simulink library "RCAM"  (R2018b)
settings: Solver=ode45  StartTime=0.0  StopTime=10.0  RelTol=1e-3  EnableMultiTasking=on
values from neighbouring files (symbols this model uses):
  a0 = 15.212    [RCAM_SS_flat_earth_wind.m]
  a1 = -155.2    [RCAM_SS_flat_earth_wind.m]
  a2 = 609.2    [RCAM_SS_flat_earth_wind.m]
  a3 = -768.5    [RCAM_SS_flat_earth_wind.m]
  alpha_L0 = -11.5*pi/180    (= -0.200712863979)    [RCAM_SS_flat_earth_wind.m]
  alpha_switch = 14.5*(pi/180)    (= 0.253072741539)    [RCAM_SS_flat_earth_wind.m]
  cbar = 6.6    [RCAM_SS_flat_earth_wind.m]
  depsda = 0.25    [RCAM_SS_flat_earth_wind.m]
  Ib = m*[40.07 0 -2.0923 ... (first row only)    [RCAM_SS_flat_earth_wind.m]
  lt = 24.8    [RCAM_SS_flat_earth_wind.m]
  m = 120000    [RCAM_SS_flat_earth_wind.m]
  n = 5.5    [RCAM_SS_flat_earth_wind.m]
  S = 260    [RCAM_SS_flat_earth_wind.m]
  St = 64    [RCAM_SS_flat_earth_wind.m]
  Umax = 120000*9.81    (= 1177200)    [RCAM_SS_flat_earth_wind.m]
  Xac = 0.12*cbar    (= 0.792)    [RCAM_SS_flat_earth_wind.m]
  Xapt1 = 0    [RCAM_SS_flat_earth_wind.m]
  Xapt2 = 0    [RCAM_SS_flat_earth_wind.m]
  Yac = 0    [RCAM_SS_flat_earth_wind.m]
  Yapt1 = -7.94    [RCAM_SS_flat_earth_wind.m]
  Yapt2 = 7.94    [RCAM_SS_flat_earth_wind.m]
  Zac = 0    [RCAM_SS_flat_earth_wind.m]
  Zapt1 = -1.9    [RCAM_SS_flat_earth_wind.m]
  Zapt2 = -1.9    [RCAM_SS_flat_earth_wind.m]
undefined symbols (not defined in the file or in its folder): RCAM_SS_flat_earth_wind, X0, Xo
libraries: UWAerospaceBlockset_Utilities x4, $bdroot x3, aerolibutil x2, aerolibobsolete x1, aerolibadyn x1, UWAerospaceBlockset_FlightParameters x1
settings Model: Creator=Christopher  LastModifiedBy=Christopher
settings DataIOCC: LimitDataPoints=on  SaveFormat=Array
settings OptimizationCC: LifeSpan=inf
settings DebuggingCC: SolverPrmCheckMsg=warning  SFUnexpectedBacktrackingDiag=warning  SFNoUnconditionalDefaultTransitionDiag=warning  SFExecutionAtInitializationDiag=none
settings HardwareCC: ProdBitPerPointer=32  ProdBitPerSizeT=32  ProdBitPerPtrDiffT=32  ProdLargestAtomicFloat=None  ProdIntDivRoundTo=Undefined  ProdEndianess=Unspecified  ProdWordSize=32  ProdHWDeviceType=32-bit Generic
settings ModelReferenceCC: PropagateSignalLabelsOutOfModel=off
settings SFSimCC: SimUseLocalCustomCode=off
settings RTWCC: RTWUseLocalCustomCode=off
settings CodeAppCC: StateflowObjectComments=on
settings GRTTargetCC: TargetLangStandard=C89/C90 (ANSI)  GeneratePreprocessorConditionals=Disable all
settings ConfigComp: CovMetricSettings=dw  CovHtmlReporting=on  CovSaveCumulativeToWorkspaceVar=on  CovSaveSingleToWorkspaceVar=on  CovExternalEMLEnable=off  CovSFcnEnable=off

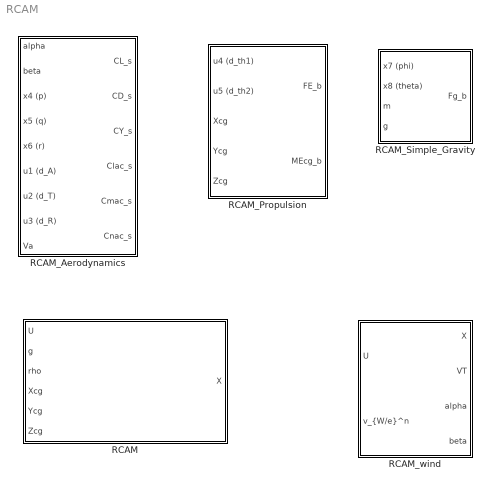
== system RCAM ==
  RCAM : Subsystem  mask{Xo=Xo, m=m, cbar=cbar, lt=lt, S=S, St=St, Xac=Xac, Yac=Yac, Zac=Zac, Umax=Umax, Xapt1=Xapt1, Yapt1=Yapt1, Zapt1=Zapt1, Xapt2=Xapt2, Yapt2=Yapt2, Zapt2=Zapt2, depsda=depsda, alpha_L0=alpha_L0, n=n, a3=a3, a2=a2, a1=a1, a0=a0, alpha_switch=alpha_switch, Ib=Ib}
      mask prompts: Xo "Xo: initial condition"; m "m: mass"; cbar "cbar: mean aerodynamic chord (m)"; lt "lt: distance bw AC of tail and body (m)"; S "S: wing planform area (m^2)"; St "St: tail planform area (m^2)"; Xac "Xac: x position of aerodynamic center in Fm (m)"; Yac "Yac: y position of aerodynamic center in Fm (m)"; Zac "Zac: z position of aerodynamic center in Fm (m)"; Umax "Umax: maximum thrust provided by one engine (N)"; Xapt1 "Xapt1: x position of engine 1 force in Fm (m)"; Yapt1 "Yapt1: y position of engine 1 force in Fm (m)"; Zapt1 "Zapt1: z position of engine 1 force in Fm (m)"; Xapt2 "Xapt2: x position of engine 2 force in Fm (m)"; Yapt2 "Yapt2: y position of engine 2 force in Fm (m)"; Zapt2 "Zapt2: z position of engine 2 force in Fm (m)"; depsda "depsda: change in downwash w.r.t. alpha (rad/rad)"; alpha_L0 "alpha_L0: zero lift angle of attack (rad)"; n "n: slope of linear region of lift slope"; alpha_switch "alpha_switch: alpha where lift slope goes from linear to non-linear"; Ib "Ib: inertia matrix"
      mask help:
      | Implements the RCAM model using Simulink blocks.
      |
      | State vector X and input vector U is defined as
      |
      |     X = [   u (m/s)
      |             v (m/s)
      |             w (m/s)
      |             p (rad/s)
      |             q (rad/s)
      |             r (rad/s)
      |             phi (bank angle: rad)
      |             theta (pitch angle: rad)
      |             psi (yaw angle: rad)
      |             P_N (position north (AKA X_e): m)
      |             P_E (position east (AKA Y_e): m)
      |             P_D (position down (AKA Z_e): m)
      |         ]
      |
      |     U = [   d_A (aileron deflection: rad)
      |             d_T (horizontal tail/elevator deflection: rad)
      |             d_R (rudder deflection: rad)
      |             d_th1 (throttle 1 deflection: in range [0,1])
      |             d_th2 (throttle 2 deflection: in range [0,1])
      |         ]
      |
      | The mass of this model is fixed but the CG location can move.
      |
      | INPUT:  U:      control vector
      |         g:      gravity magnitude (typically 9.81)
      |         rho:    density (kg/m^3)
      |         Xcg:    x position of CG (m)
      |         Ycg:    y position of CG (m)
      |         Zcg:    z position of CG (m)
      |
      | OUTPUT: X:      state vector
      |
      | Christopher Lum
      | lum@uw.edu
      mask Display: image('RCAM_icon.jpg')
  RCAM_Aerodynamics : Subsystem  mask{depsda=0.25, alpha_L0=-11.5*pi/180, n=5.5, a3=-768.5, a2=609.2, a1=-155.2, a0=15.2, alpha_switch=14.5*(pi/180), cbar=6.6, lt=24.8, S=260, St=64}
      mask prompts: depsda "depsda: change in downwash w.r.t. alpha (rad/rad)"; alpha_L0 "alpha_L0: zero lift angle of attack (rad)"; n "n: slope of linear region of lift slope"; alpha_switch "alpha_switch: alpha where lift slope goes from linear to non-linear (rad)"; cbar "cbar: mean aerodynamic chord"; lt "lt: distance between AC of tail and body"; S "S: wing planform area"; St "St: tail planform area"
      mask help:
      | Compute aerodynamic moment coefficients for the RCAM model.
      |
      | INPUT:  self explantory
      |
      | OUTPUT: force and moment coefficients such that the normalized values are expressed in the stability axis
  RCAM_Propulsion : Subsystem  mask{Umax=120000*9.81, Xapt1=0, Yapt1=-7.94, Zapt1=-1.9, Xapt2=0, Yapt2=7.94, Zapt2=-1.9}
      mask prompts: Umax "Umax (maximum engine thrust, same value applied to both engine 1 and 2)"; Xapt1 "Xapt1 (x position of engine 1 force in Fm)"; Yapt1 "Yapt1 (y position of engine 1 force in Fm)"; Zapt1 "Zapt1 (z position of engine 1 force in Fm)"; Xapt2 "Xapt2 (x position of engine 2 force in Fm)"; Yapt2 "Yapt2 (y position of engine 2 force in Fm)"; Zapt2 "Zapt2 (z position of engine 2 force in Fm)"
      mask help:
      | Calculates propulsion forces and moments for RCAM model.
      |
      | INPUT:  u4 (d_th1): throttle position 1
      |         u4 (d_th2): throttle position 2
      |         Xcg:        x location of CG
      |         Ycg:        y location of CG
      |         Zcg:        z location of CG
      |
      | OUTPUT: FE_b:       engine force vector expressed in body frame
      |         MEcg_b:     engine moment about CG expressed in body frame
  RCAM_Simple_Gravity : Subsystem
      mask help:
      | Computes the gravitational force in the body frame using the simple relationship of
      |
      | Fg_b = m*g*[-sin(x8);cos(x8)*sin(x7); cos(x8)*cos(x7)]
      |
      | INPUT:  x7 (phi):   bank Euler angle
      |         x8 (theta): pitch Euler angle
      |         m:          mass
      |         g:          gravitational acceleration
      |
      | OUTPUT: Fg_b:       gravitational force in body frame
  RCAM_wind : Subsystem  mask{Xo=X0}
      mask prompts: Xo "Xo: initial condition"
      mask help:
      | Implements the RCAM model with nominal constants with constant wind.
      |
      | State vector X and input vector U is defined as
      |
      |     X = [   u (m/s)
      |             v (m/s)
      |             w (m/s)
      |             p (rad/s)
      |             q (rad/s)
      |             r (rad/s)
      |             phi (bank angle: rad)
      |             theta (pitch angle: rad)
      |             psi (yaw angle: rad)
      |             P_N (position north (AKA X_e): m)
      |             P_E (position east (AKA Y_e): m)
      |             P_D (position down (AKA Z_e): m)
      |         ]
      |
      |     U = [   d_A (aileron deflection: rad)
      |             d_T (horizontal tail/elevator deflection: rad)
      |             d_R (rudder deflection: rad)
      |             d_th1 (throttle 1 deflection: in range [0,1])
      |             d_th2 (throttle 2 deflection: in range [0,1])
      |         ]
      |
      | The wind vector is defined as
      |
      |     v_{W/e}^n = [W_N; W_E; W_D]
      |
      | INPUT:  U:          control vector
      |         v_{W/e}^n:  3x1 wind vector
      |
      | OUTPUT: X:          state vector

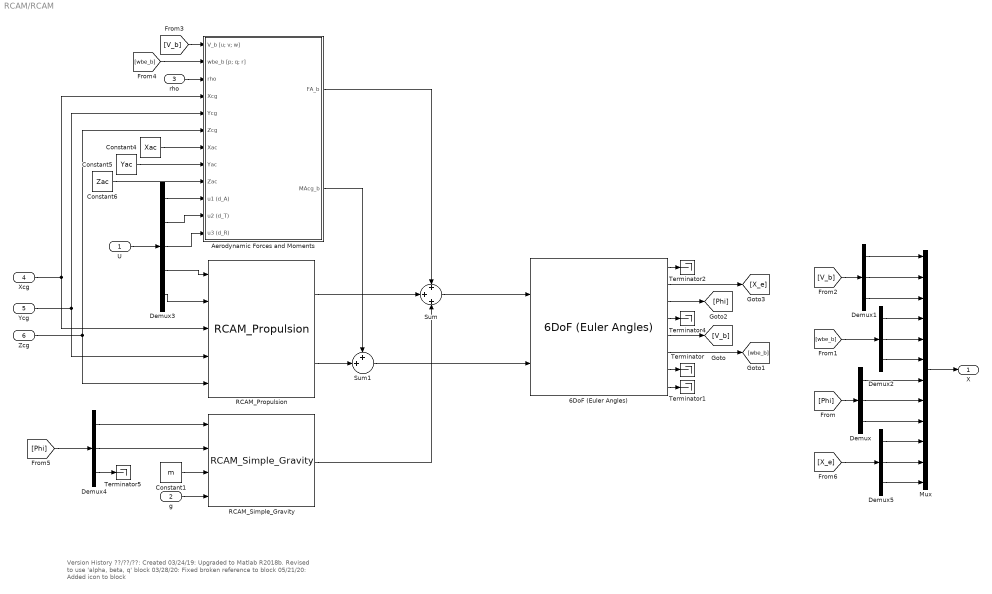
== system RCAM/RCAM ==
  note: Version History
      | ??/??/??: Created
      | 03/24/19: Upgraded to Matlab R2018b.  Revised to use 'alpha, beta, q' block
      | 03/28/20: Fixed broken reference to block
      | 05/21/20: Added icon to block
  U : Inport
  g : Inport  Port=2
  rho : Inport  Port=3
  Xcg : Inport  Port=4
  Ycg : Inport  Port=5
  Zcg : Inport  Port=6
  6DoF (Euler Angles) : aerolibobsolete/6DoF (Euler Angles)  units=Metric (MKS)  mtype=Fixed  rep=Euler Angles  xme_0=Xo(10:12)  Vm_0=Xo(1:3)  eul_0=Xo(7:9)  pm_0=Xo(4:6)  mass_0=m  mass_e=0.5  mass_f=2.0  inertia=Ib  inertia_e=eye(3)  inertia_f=2*eye(3)  k_quat=1.0
      settings: SourceProductName=Aerospace Blockset  SourceProductBaseCode=AE
  Aerodynamic Forces and Moments : Subsystem
  Constant1 : Constant  Value=m
  Constant4 : Constant  Value=Xac
  Constant5 : Constant  Value=Yac
  Constant6 : Constant  Value=Zac
  Demux{,1..2,4..5} (5 alike) : Demux  Outputs=3
  Demux3 : Demux  Outputs=5
  Mux : Mux  Inputs=12
  RCAM_Propulsion : $bdroot/RCAM_Propulsion  Umax=Umax  Xapt1=Xapt1  Yapt1=Yapt1  Zapt1=Zapt1  Xapt2=Xapt2  Yapt2=Yapt2  Zapt2=Zapt2
  RCAM_Simple_Gravity : $bdroot/RCAM_Simple_Gravity
  Sum : Sum  Inputs=+|+|+
  Sum1 : Sum  Inputs=++|
  Terminator{,1..2,4..5} (5 alike) : Terminator
  X : Outport
  wires:
  Aerodynamic Forces and Moments/1(FA_b) -> Sum/1
  RCAM_Propulsion/1 -> Sum/2
  RCAM_Simple_Gravity/1 -> Sum/3
  Aerodynamic Forces and Moments/2(MAcg_b) -> Sum1/1
  RCAM_Propulsion/2 -> Sum1/2
  Sum/1 -> 6DoF (Euler Angles)/1
  Sum1/1 -> 6DoF (Euler Angles)/2
  Demux/1 -> Mux/7
  Demux/2 -> Mux/8
  Demux/3 -> Mux/9
  Demux1/1 -> Mux/1
  Demux1/2 -> Mux/2
  Demux1/3 -> Mux/3
  Demux2/1 -> Mux/4
  Demux2/2 -> Mux/5
  Demux2/3 -> Mux/6
  6DoF (Euler Angles)/7 -> Terminator/1
  6DoF (Euler Angles)/8 -> Terminator1/1
  6DoF (Euler Angles)/1 -> Terminator2/1
  6DoF (Euler Angles)/2 -> [X_e]
  6DoF (Euler Angles)/4 -> Terminator4/1
  Mux/1 -> X/1
  6DoF (Euler Angles)/5 -> [V_b]
  6DoF (Euler Angles)/6 -> [wbe_b]
  6DoF (Euler Angles)/3 -> [Phi]
  [Phi] -> Demux/1
  [wbe_b] -> Demux2/1
  [V_b] -> Demux1/1
  rho/1 -> Aerodynamic Forces and Moments/3(rho)
  [V_b] -> Aerodynamic Forces and Moments/1(V_b [u; v; w])
  [wbe_b] -> Aerodynamic Forces and Moments/2(wbe_b [p; q; r])
  Constant4/1 -> Aerodynamic Forces and Moments/7(Xac)
  Constant5/1 -> Aerodynamic Forces and Moments/8(Yac)
  Constant6/1 -> Aerodynamic Forces and Moments/9(Zac)
  Demux3/1 -> Aerodynamic Forces and Moments/10(u1 (d_A))
  Demux3/2 -> Aerodynamic Forces and Moments/11(u2 (d_T))
  Demux3/3 -> Aerodynamic Forces and Moments/12(u3 (d_R))
  U/1 -> Demux3/1
  Demux3/4 -> RCAM_Propulsion/1
  Demux3/5 -> RCAM_Propulsion/2
  [Phi] -> Demux4/1
  Demux4/1 -> RCAM_Simple_Gravity/1
  Demux4/2 -> RCAM_Simple_Gravity/2
  Demux4/3 -> Terminator5/1
  Constant1/1 -> RCAM_Simple_Gravity/3
  g/1 -> RCAM_Simple_Gravity/4
  Xcg/1 -> RCAM_Propulsion/3, Aerodynamic Forces and Moments/4(Xcg)
  Ycg/1 -> RCAM_Propulsion/4, Aerodynamic Forces and Moments/5(Ycg)
  Zcg/1 -> RCAM_Propulsion/5, Aerodynamic Forces and Moments/6(Zcg)
  [X_e] -> Demux5/1
  Demux5/3 -> Mux/12
  Demux5/1 -> Mux/10
  Demux5/2 -> Mux/11

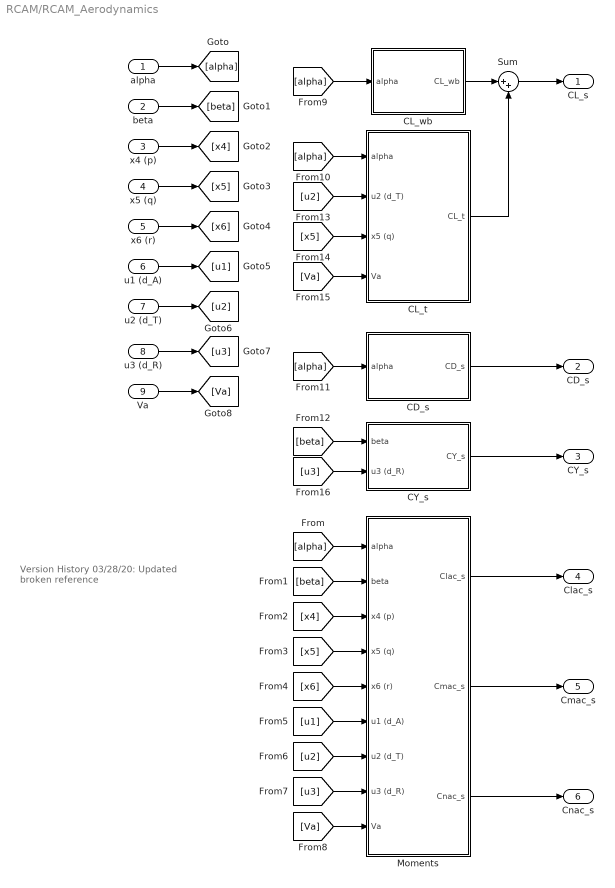
== system RCAM/RCAM_Aerodynamics ==
  note: Version History
      | 03/28/20: Updated broken reference
  alpha : Inport
  beta : Inport  Port=2
  x4 (p) : Inport  Port=3
  x5 (q) : Inport  Port=4
  x6 (r) : Inport  Port=5
  u1 (d_A) : Inport  Port=6
  u2 (d_T) : Inport  Port=7
  u3 (d_R) : Inport  Port=8
  Va : Inport  Port=9
  "CD_s " : Subsystem
  CL_t : Subsystem
  CL_wb : Subsystem
  "CY_s " : Subsystem
  Moments : Subsystem
  Sum : Sum  Inputs=|++
  CL_s : Outport
  CD_s : Outport  Port=2
  CY_s : Outport  Port=3
  Clac_s : Outport  Port=4
  Cmac_s : Outport  Port=5
  Cnac_s : Outport  Port=6
  wires:
  CL_wb/1(CL_wb) -> Sum/1
  CL_t/1(CL_t) -> Sum/2
  Sum/1 -> CL_s/1
  "CD_s "/1(CD_s) -> CD_s/1
  "CY_s "/1(CY_s) -> CY_s/1
  Moments/1(Clac_s) -> Clac_s/1
  Moments/2(Cmac_s) -> Cmac_s/1
  Moments/3(Cnac_s) -> Cnac_s/1
  alpha/1 -> [alpha]
  beta/1 -> [beta]
  x4 (p)/1 -> [x4]
  x5 (q)/1 -> [x5]
  x6 (r)/1 -> [x6]
  u1 (d_A)/1 -> [u1]
  u2 (d_T)/1 -> [u2]
  u3 (d_R)/1 -> [u3]
  Va/1 -> [Va]
  [alpha] -> Moments/1(alpha)
  [beta] -> Moments/2(beta)
  [x4] -> Moments/3(x4 (p))
  [x5] -> Moments/4(x5 (q))
  [x6] -> Moments/5(x6 (r))
  [u1] -> Moments/6(u1 (d_A))
  [u2] -> Moments/7(u2 (d_T))
  [u3] -> Moments/8(u3 (d_R))
  [Va] -> Moments/9(Va)
  [alpha] -> CL_wb/1(alpha)
  [alpha] -> CL_t/1(alpha)
  [alpha] -> "CD_s "/1(alpha)
  [beta] -> "CY_s "/1(beta)
  [u2] -> CL_t/2(u2 (d_T))
  [x5] -> CL_t/3(x5 (q))
  [Va] -> CL_t/4(Va)
  [u3] -> "CY_s "/2(u3 (d_R))

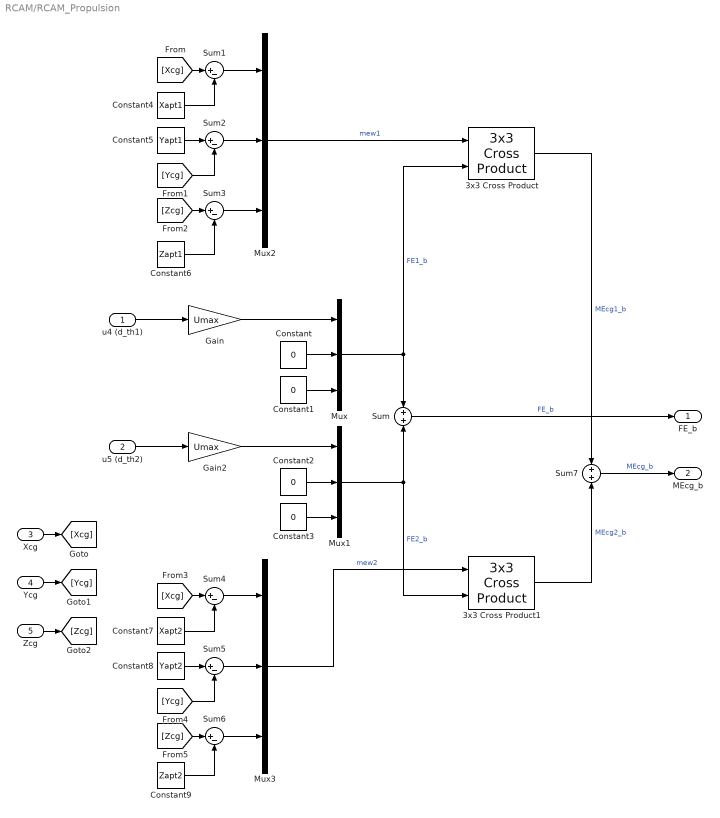
== system RCAM/RCAM_Propulsion ==
  u4 (d_th1) : Inport
  u5 (d_th2) : Inport  Port=2
  Xcg : Inport  Port=3
  Ycg : Inport  Port=4
  Zcg : Inport  Port=5
  3x3 Cross Product : aerolibutil/3x3 Cross Product
      settings: SourceProductName=Aerospace Blockset  SourceProductBaseCode=AE
  3x3 Cross Product1 : aerolibutil/3x3 Cross Product
      settings: SourceProductName=Aerospace Blockset  SourceProductBaseCode=AE
  Constant{,1..3} (4 alike) : Constant  Value=0
  Constant4 : Constant  Value=Xapt1
  Constant5 : Constant  Value=Yapt1
  Constant6 : Constant  Value=Zapt1
  Constant7 : Constant  Value=Xapt2
  Constant8 : Constant  Value=Yapt2
  Constant9 : Constant  Value=Zapt2
  Gain : Gain  Gain=Umax
  Gain2 : Gain  Gain=Umax
  Mux{,1..3} (4 alike) : Mux  Inputs=3
  Sum : Sum  Inputs=+|+
  Sum{1..6} (6 alike) : Sum  Inputs=|+-
  Sum7 : Sum  Inputs=+|+
  FE_b : Outport
  MEcg_b : Outport  Port=2
  wires:
  u4 (d_th1)/1 -> Gain/1
  u5 (d_th2)/1 -> Gain2/1
  Constant/1 -> Mux/2
  Constant1/1 -> Mux/3
  Gain/1 -> Mux/1
  Mux/1 -> Sum/1, 3x3 Cross Product/2  "FE1_b"
  Constant2/1 -> Mux1/2
  Constant3/1 -> Mux1/3
  Gain2/1 -> Mux1/1
  Mux1/1 -> Sum/2, 3x3 Cross Product1/2  "FE2_b"
  Constant4/1 -> Sum1/2
  Sum1/1 -> Mux2/1
  Constant5/1 -> Sum2/1
  Sum2/1 -> Mux2/2
  Constant6/1 -> Sum3/2
  Sum3/1 -> Mux2/3
  Xcg/1 -> [Xcg]
  Ycg/1 -> [Ycg]
  Zcg/1 -> [Zcg]
  [Xcg] -> Sum1/1
  [Ycg] -> Sum2/2
  [Zcg] -> Sum3/1
  Constant7/1 -> Sum4/2
  Sum4/1 -> Mux3/1
  Constant8/1 -> Sum5/1
  Sum5/1 -> Mux3/2
  Constant9/1 -> Sum6/2
  Sum6/1 -> Mux3/3
  [Xcg] -> Sum4/1
  [Ycg] -> Sum5/2
  [Zcg] -> Sum6/1
  Mux2/1 -> 3x3 Cross Product/1  "mew1"
  Mux3/1 -> 3x3 Cross Product1/1  "mew2"
  Sum/1 -> FE_b/1  "FE_b"
  3x3 Cross Product/1 -> Sum7/1  "MEcg1_b"
  3x3 Cross Product1/1 -> Sum7/2  "MEcg2_b"
  Sum7/1 -> MEcg_b/1  "MEcg_b"

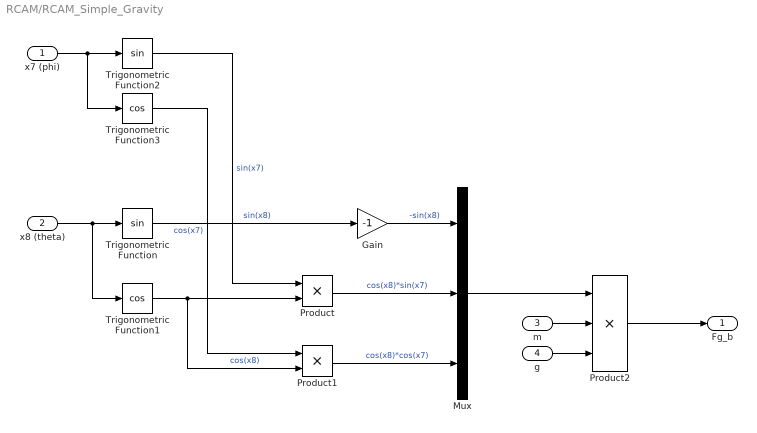
== system RCAM/RCAM_Simple_Gravity ==
  x7 (phi) : Inport
  x8 (theta) : Inport  Port=2
  m : Inport  Port=3
  g : Inport  Port=4
  Gain : Gain  Gain=-1
  Mux : Mux  Inputs=3
  Product : Product  RndMeth=Zero
  Product1 : Product  RndMeth=Zero
  Product2 : Product  Inputs=3  RndMeth=Zero
  Trigonometric Function : Trigonometry
  Trigonometric Function1 : Trigonometry  Operator=cos
  Trigonometric Function2 : Trigonometry
  Trigonometric Function3 : Trigonometry  Operator=cos
  Fg_b : Outport
  wires:
  Mux/1 -> Product2/1
  x8 (theta)/1 -> Trigonometric Function/1, Trigonometric Function1/1
  Trigonometric Function/1 -> Gain/1  "sin(x8)"
  Trigonometric Function1/1 -> Product/2, Product1/2  "cos(x8)"
  x7 (phi)/1 -> Trigonometric Function2/1, Trigonometric Function3/1
  Trigonometric Function2/1 -> Product/1  "sin(x7)"
  Trigonometric Function3/1 -> Product1/1  "cos(x7)"
  Gain/1 -> Mux/1  "-sin(x8)"
  Product/1 -> Mux/2  "cos(x8)*sin(x7)"
  Product1/1 -> Mux/3  "cos(x8)*cos(x7)"
  m/1 -> Product2/2
  g/1 -> Product2/3
  Product2/1 -> Fg_b/1

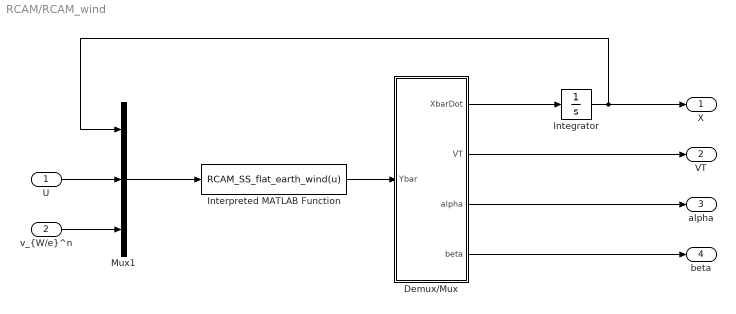
== system RCAM/RCAM_wind ==
  U : Inport
  "v_{W/e}^n" : Inport  Port=2
  Demux/Mux : Subsystem
  Integrator : Integrator  InitialCondition=X0
  Interpreted MATLAB Function : MATLABFcn  MATLABFcn=RCAM_SS_flat_earth_wind(u)  OutputDimensions=12+3
  Mux1 : Mux  Inputs=3
  X : Outport
  VT : Outport  Port=2
  alpha : Outport  Port=3
  beta : Outport  Port=4
  wires:
  Interpreted MATLAB Function/1 -> Demux/Mux/1(Ybar)
  Mux1/1 -> Interpreted MATLAB Function/1
  Demux/Mux/1(XbarDot) -> Integrator/1
  Integrator/1 -> Mux1/1, X/1
  U/1 -> Mux1/2
  "v_{W/e}^n"/1 -> Mux1/3
  Demux/Mux/2(VT) -> VT/1
  Demux/Mux/3(alpha) -> alpha/1
  Demux/Mux/4(beta) -> beta/1

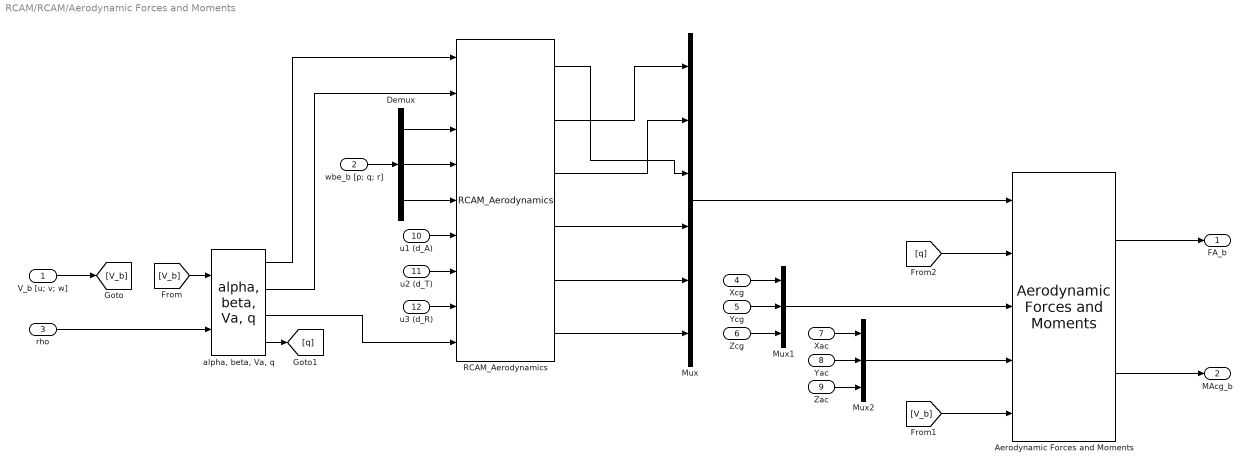
== system RCAM/RCAM/Aerodynamic Forces and Moments ==
  V_b [u; v; w] : Inport
  wbe_b [p; q; r] : Inport  Port=2
  rho : Inport  Port=3
  Xcg : Inport  Port=4
  Ycg : Inport  Port=5
  Zcg : Inport  Port=6
  Xac : Inport  Port=7
  Yac : Inport  Port=8
  Zac : Inport  Port=9
  u1 (d_A) : Inport  Port=10
  u2 (d_T) : Inport  Port=11
  u3 (d_R) : Inport  Port=12
  "Aerodynamic Forces and Moments " : aerolibadyn/Aerodynamic Forces and Moments   inputAxes=Stability  outputForceAxes=Body  outputMomentAxes=Body  S=S  b=cbar  cbar=cbar
      settings: SourceProductName=Aerospace Blockset
  Demux : Demux  Outputs=3
  Mux : Mux  Inputs=6
  Mux1 : Mux  Inputs=3
  Mux2 : Mux  Inputs=3
  RCAM_Aerodynamics : $bdroot/RCAM_Aerodynamics  depsda=depsda  alpha_L0=alpha_L0  n=n  a3=a3  a2=a2  a1=a1  a0=a0  alpha_switch=alpha_switch  cbar=cbar  lt=lt  S=S  St=St
  "alpha, beta, Va, q" : UWAerospaceBlockset_FlightParameters/alpha, beta, Va, q
  FA_b : Outport
  MAcg_b : Outport  Port=2
  wires:
  Mux/1 -> "Aerodynamic Forces and Moments "/1
  RCAM_Aerodynamics/4 -> Mux/4
  RCAM_Aerodynamics/5 -> Mux/5
  RCAM_Aerodynamics/6 -> Mux/6
  RCAM_Aerodynamics/2 -> Mux/1
  RCAM_Aerodynamics/3 -> Mux/2
  RCAM_Aerodynamics/1 -> Mux/3
  V_b [u; v; w]/1 -> [V_b]
  [V_b] -> "alpha, beta, Va, q"/1
  rho/1 -> "alpha, beta, Va, q"/2
  [V_b] -> "Aerodynamic Forces and Moments "/5
  Mux1/1 -> "Aerodynamic Forces and Moments "/3
  Mux2/1 -> "Aerodynamic Forces and Moments "/4
  Xac/1 -> Mux2/1
  Yac/1 -> Mux2/2
  Zac/1 -> Mux2/3
  [q] -> "Aerodynamic Forces and Moments "/2
  u1 (d_A)/1 -> RCAM_Aerodynamics/6
  u2 (d_T)/1 -> RCAM_Aerodynamics/7
  u3 (d_R)/1 -> RCAM_Aerodynamics/8
  "alpha, beta, Va, q"/1 -> RCAM_Aerodynamics/1
  "alpha, beta, Va, q"/2 -> RCAM_Aerodynamics/2
  Demux/1 -> RCAM_Aerodynamics/3
  Demux/2 -> RCAM_Aerodynamics/4
  Demux/3 -> RCAM_Aerodynamics/5
  wbe_b [p; q; r]/1 -> Demux/1
  "Aerodynamic Forces and Moments "/1 -> FA_b/1
  "Aerodynamic Forces and Moments "/2 -> MAcg_b/1
  Xcg/1 -> Mux1/1
  Ycg/1 -> Mux1/2
  Zcg/1 -> Mux1/3
  "alpha, beta, Va, q"/4 -> [q]
  "alpha, beta, Va, q"/3 -> RCAM_Aerodynamics/9

== system RCAM/RCAM_Aerodynamics/CD_s  ==
  alpha : Inport
  Fcn : Fcn  Expr=0.13 + 0.07*(5.5*u + 0.654)^2
  CD_s : Outport
  wires:
  alpha/1 -> Fcn/1
  Fcn/1 -> CD_s/1

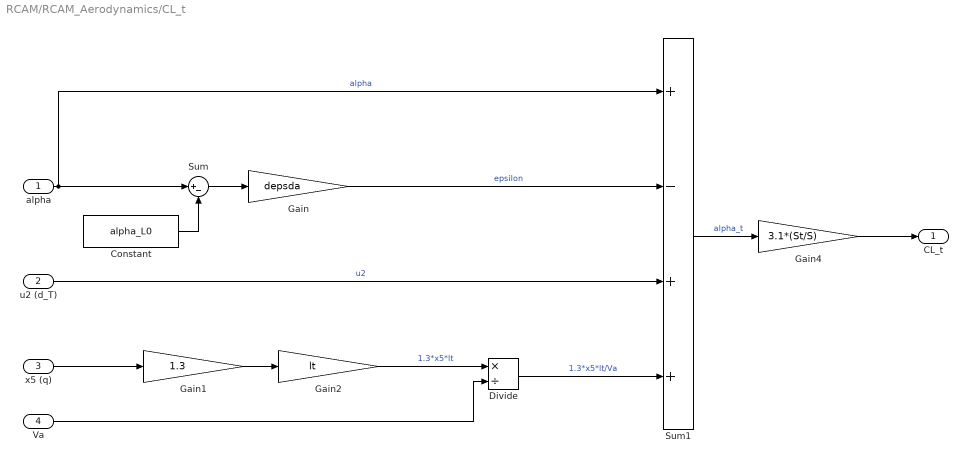
== system RCAM/RCAM_Aerodynamics/CL_t ==
  alpha : Inport
  u2 (d_T) : Inport  Port=2
  x5 (q) : Inport  Port=3
  Va : Inport  Port=4
  Constant : Constant  Value=alpha_L0
  Divide : Product  Inputs=*/
  Gain : Gain  Gain=depsda
  Gain1 : Gain  Gain=1.3
  Gain2 : Gain  Gain=lt
  Gain4 : Gain  Gain=3.1*(St/S)
  Sum : Sum  Inputs=|+-
  Sum1 : Sum  Inputs=+-++
  CL_t : Outport
  wires:
  Sum/1 -> Gain/1
  Constant/1 -> Sum/2
  alpha/1 -> Sum/1, Sum1/1  "alpha"
  Gain/1 -> Sum1/2  "epsilon"
  u2 (d_T)/1 -> Sum1/3  "u2"
  Va/1 -> Divide/2
  x5 (q)/1 -> Gain1/1
  Gain1/1 -> Gain2/1
  Gain2/1 -> Divide/1  "1.3*x5*lt"
  Divide/1 -> Sum1/4  "1.3*x5*lt/Va"
  Sum1/1 -> Gain4/1  "alpha_t"
  Gain4/1 -> CL_t/1

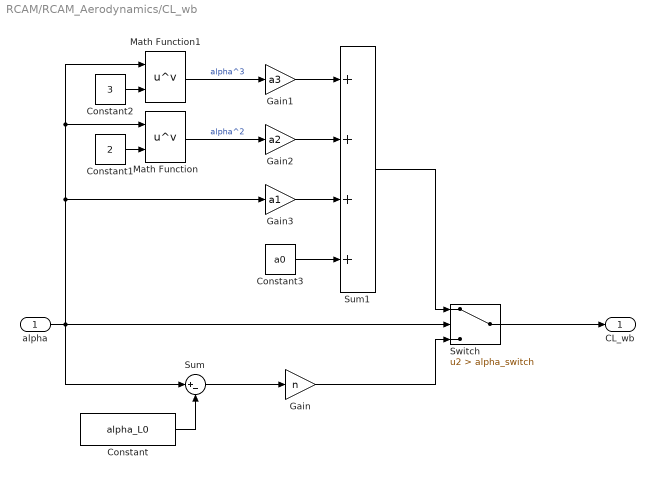
== system RCAM/RCAM_Aerodynamics/CL_wb ==
  alpha : Inport
  Constant : Constant  Value=alpha_L0
  Constant1 : Constant  Value=2
  Constant2 : Constant  Value=3
  Constant3 : Constant  Value=a0
  Gain : Gain  Gain=n
  Gain1 : Gain  Gain=a3
  Gain2 : Gain  Gain=a2
  Gain3 : Gain  Gain=a1
  Math Function : Math  Operator=pow  SaturateOnIntegerOverflow=on
  Math Function1 : Math  Operator=pow  SaturateOnIntegerOverflow=on
  Sum : Sum  Inputs=|+-
  Sum1 : Sum  Inputs=++++
  Switch : Switch  Criteria=u2 > Threshold  Threshold=alpha_switch
  CL_wb : Outport
  wires:
  Switch/1 -> CL_wb/1
  alpha/1 -> Switch/2, Sum/1, Math Function/1, Math Function1/1, Gain3/1
  Constant/1 -> Sum/2
  Sum/1 -> Gain/1
  Gain/1 -> Switch/3
  Math Function/1 -> Gain2/1  "alpha^2"
  Constant1/1 -> Math Function/2
  Constant2/1 -> Math Function1/2
  Math Function1/1 -> Gain1/1  "alpha^3"
  Gain1/1 -> Sum1/1
  Gain2/1 -> Sum1/2
  Gain3/1 -> Sum1/3
  Constant3/1 -> Sum1/4
  Sum1/1 -> Switch/1

== system RCAM/RCAM_Aerodynamics/CY_s  ==
  beta : Inport
  u3 (d_R) : Inport  Port=2
  Gain : Gain  Gain=-1.6
  Gain1 : Gain  Gain=0.24
  Sum : Sum  Inputs=|++
  CY_s : Outport
  wires:
  beta/1 -> Gain/1
  u3 (d_R)/1 -> Gain1/1
  Gain/1 -> Sum/1
  Gain1/1 -> Sum/2
  Sum/1 -> CY_s/1

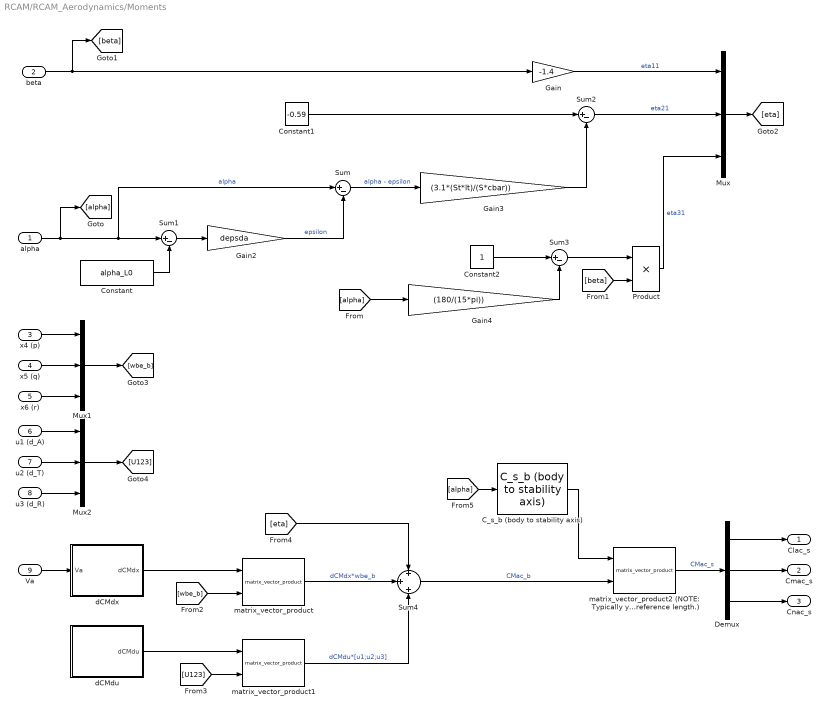
== system RCAM/RCAM_Aerodynamics/Moments ==
  alpha : Inport
  beta : Inport  Port=2
  x4 (p) : Inport  Port=3
  x5 (q) : Inport  Port=4
  x6 (r) : Inport  Port=5
  u1 (d_A) : Inport  Port=6
  u2 (d_T) : Inport  Port=7
  u3 (d_R) : Inport  Port=8
  Va : Inport  Port=9
  C_s_b (body to stability axis) : UWAerospaceBlockset_Utilities/C_s_b (body to stability axis)
  Constant : Constant  Value=alpha_L0
  Constant1 : Constant  Value=-0.59
  Constant2 : Constant
  Demux : Demux  Outputs=3
  Gain : Gain  Gain=-1.4
  Gain2 : Gain  Gain=depsda
  Gain3 : Gain  Gain=(3.1*(St*lt)/(S*cbar))
  Gain4 : Gain  Gain=(180/(15*pi))
  Mux : Mux  Inputs=3
  Mux1 : Mux  Inputs=3
  Mux2 : Mux  Inputs=3
  Product : Product  RndMeth=Zero
  Sum{,1..3} (4 alike) : Sum  Inputs=|+-
  Sum4 : Sum  Inputs=+|+|+
  dCMdu : Subsystem
  dCMdx : Subsystem
  matrix_vector_product : UWAerospaceBlockset_Utilities/matrix_vector_product
  matrix_vector_product1 : UWAerospaceBlockset_Utilities/matrix_vector_product
  matrix_vector_product2 (NOTE:  Typically you would have to renormalize coefficients to moment before applying rotation matrix. We can do this here because all moment are normalized by the same reference length.) : UWAerospaceBlockset_Utilities/matrix_vector_product
  Clac_s : Outport
  Cmac_s : Outport  Port=2
  Cnac_s : Outport  Port=3
  wires:
  beta/1 -> Gain/1, [beta]
  Gain/1 -> Mux/1  "eta11"
  Sum1/1 -> Gain2/1
  Constant/1 -> Sum1/2
  alpha/1 -> Sum1/1, Sum/1, [alpha]  "alpha"
  Gain2/1 -> Sum/2  "epsilon"
  Sum/1 -> Gain3/1  "alpha - epsilon"
  Constant1/1 -> Sum2/1
  Gain3/1 -> Sum2/2
  Sum2/1 -> Mux/2  "eta21"
  Constant2/1 -> Sum3/1
  [alpha] -> Gain4/1
  Gain4/1 -> Sum3/2
  Sum3/1 -> Product/1
  [beta] -> Product/2
  Product/1 -> Mux/3  "eta31"
  Mux/1 -> [eta]
  dCMdx/1(dCMdx) -> matrix_vector_product/1
  Va/1 -> dCMdx/1(Va)
  x4 (p)/1 -> Mux1/1
  x5 (q)/1 -> Mux1/2
  x6 (r)/1 -> Mux1/3
  Mux1/1 -> [wbe_b]
  u1 (d_A)/1 -> Mux2/1
  u2 (d_T)/1 -> Mux2/2
  u3 (d_R)/1 -> Mux2/3
  [wbe_b] -> matrix_vector_product/2
  dCMdu/1(dCMdu) -> matrix_vector_product1/1
  Mux2/1 -> [U123]
  [U123] -> matrix_vector_product1/2
  [eta] -> Sum4/1
  matrix_vector_product/1 -> Sum4/2  "dCMdx*wbe_b"
  matrix_vector_product1/1 -> Sum4/3  "dCMdu*[u1;u2;u3]"
  Sum4/1 -> matrix_vector_product2 (NOTE:  Typically you would have to renormalize coefficients to moment before applying rotation matrix. We can do this here because all moment are normalized by the same reference length.)/2  "CMac_b"
  C_s_b (body to stability axis)/1 -> matrix_vector_product2 (NOTE:  Typically you would have to renormalize coefficients to moment before applying rotation matrix. We can do this here because all moment are normalized by the same reference length.)/1
  matrix_vector_product2 (NOTE:  Typically you would have to renormalize coefficients to moment before applying rotation matrix. We can do this here because all moment are normalized by the same reference length.)/1 -> Demux/1  "CMac_s"
  [alpha] -> C_s_b (body to stability axis)/1
  Demux/1 -> Clac_s/1
  Demux/2 -> Cmac_s/1
  Demux/3 -> Cnac_s/1

== system RCAM/RCAM_wind/Demux//Mux ==
  Ybar : Inport
  Demux : Demux  Outputs=12+3
  Mux1 : Mux  Inputs=12
  XbarDot : Outport
  VT : Outport  Port=2
  alpha : Outport  Port=3
  beta : Outport  Port=4
  wires:
  Demux/13 -> VT/1
  Demux/15 -> beta/1
  Ybar/1 -> Demux/1
  Demux/14 -> alpha/1
  Mux1/1 -> XbarDot/1
  Demux/11 -> Mux1/11
  Demux/9 -> Mux1/9
  Demux/12 -> Mux1/12
  Demux/10 -> Mux1/10
  Demux/8 -> Mux1/8
  Demux/6 -> Mux1/6
  Demux/7 -> Mux1/7
  Demux/2 -> Mux1/2
  Demux/5 -> Mux1/5
  Demux/4 -> Mux1/4
  Demux/3 -> Mux1/3
  Demux/1 -> Mux1/1

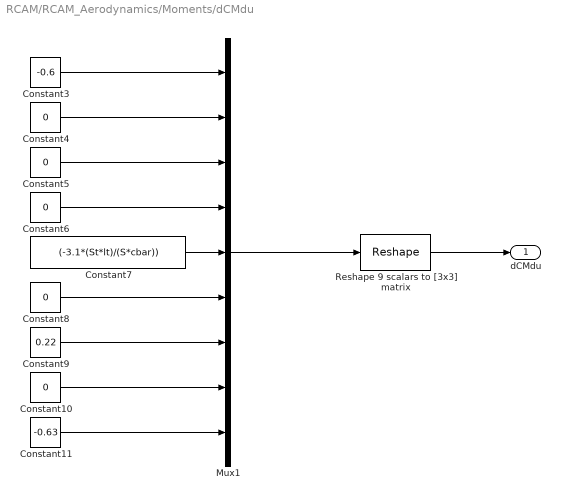
== system RCAM/RCAM_Aerodynamics/Moments/dCMdu ==
  Constant{4..6,8,10} (5 alike) : Constant  Value=0
  Constant11 : Constant  Value=-0.63
  Constant3 : Constant  Value=-0.6
  Constant7 : Constant  Value=(-3.1*(St*lt)/(S*cbar))
  Constant9 : Constant  Value=0.22
  Mux1 : Mux  Inputs=9
  Reshape 9 scalars to [3x3] matrix : Reshape  OutputDimensionality=Customize  OutputDimensions=[3,3]
  dCMdu : Outport
  wires:
  Reshape 9 scalars to [3x3] matrix/1 -> dCMdu/1
  Constant11/1 -> Mux1/9
  Constant10/1 -> Mux1/8
  Constant9/1 -> Mux1/7
  Constant8/1 -> Mux1/6
  Constant7/1 -> Mux1/5
  Constant6/1 -> Mux1/4
  Constant5/1 -> Mux1/3
  Constant4/1 -> Mux1/2
  Constant3/1 -> Mux1/1
  Mux1/1 -> Reshape 9 scalars to [3x3] matrix/1

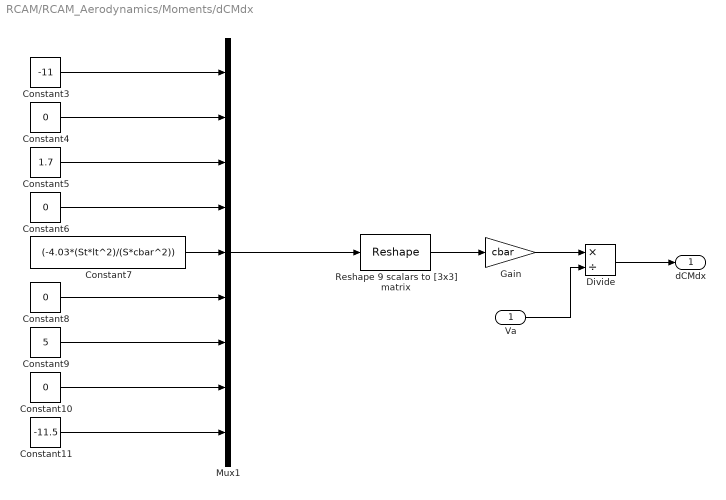
== system RCAM/RCAM_Aerodynamics/Moments/dCMdx ==
  Va : Inport
  Constant{4,6,8,10} (4 alike) : Constant  Value=0
  Constant11 : Constant  Value=-11.5
  Constant3 : Constant  Value=-11
  Constant5 : Constant  Value=1.7
  Constant7 : Constant  Value=(-4.03*(St*lt^2)/(S*cbar^2))
  Constant9 : Constant  Value=5
  Divide : Product  Inputs=*/
  Gain : Gain  Gain=cbar
  Mux1 : Mux  Inputs=9
  Reshape 9 scalars to [3x3] matrix : Reshape  OutputDimensionality=Customize  OutputDimensions=[3,3]
  dCMdx : Outport
  wires:
  Mux1/1 -> Reshape 9 scalars to [3x3] matrix/1
  Constant3/1 -> Mux1/1
  Constant4/1 -> Mux1/2
  Constant5/1 -> Mux1/3
  Constant6/1 -> Mux1/4
  Constant7/1 -> Mux1/5
  Constant8/1 -> Mux1/6
  Constant9/1 -> Mux1/7
  Constant10/1 -> Mux1/8
  Constant11/1 -> Mux1/9
  Reshape 9 scalars to [3x3] matrix/1 -> Gain/1
  Gain/1 -> Divide/1
  Va/1 -> Divide/2
  Divide/1 -> dCMdx/1
